simulink model "SS6_feb12"  (R2014b)
settings: Solver=ode3  StartTime=0.0  StopTime=40  FixedStep=0.001  RelTol=1e-3
undefined symbols (not defined in the file): INOP
libraries: simulink x1
settings Model: Creator=Bismaya  LastModifiedBy=Bismaya

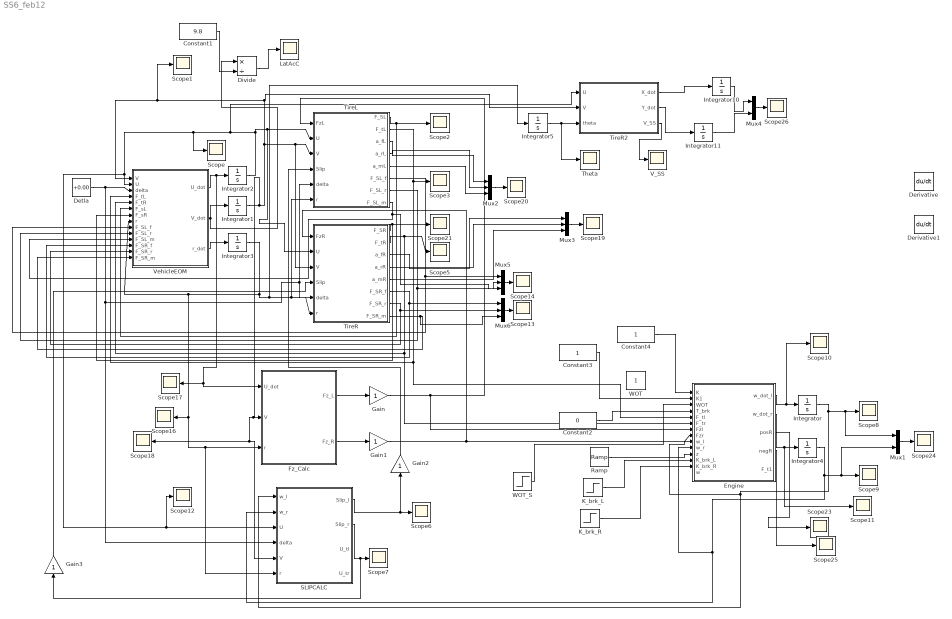
== system SS6_feb12 ==
  Constant1 : Constant  Value=9.8
  Constant2 : Constant  Value=0
  Constant3 : Constant
  Constant4 : Constant
  Derivative : Derivative
  Derivative1 : Derivative
  Detla : Constant  Value=+0.00
  Divide : Product  Inputs=*/
  Engine : MATLAB Function  TreatAsAtomicUnit=on
  Fz_Calc : MATLAB Function  TreatAsAtomicUnit=on
  Gain{,1..3} (4 alike) : Gain
  Integrator : Integrator  InitialCondition=12  LowerSaturationLimit=-0.0001
  Integrator{1,3,5,10..11} (5 alike) : Integrator
  Integrator2 : Integrator  InitialCondition=10/3
  Integrator4 : Integrator  InitialCondition=12  LowerSaturationLimit=-0.0001
  K_brk_L : Step  Time=0  After=0  SampleTime=0
  K_brk_R : Step  Time=20  After=INOP  SampleTime=0
  LatAcC : Scope
      settings: YMin=-2e-06  YMax=6e-06  SaveName=V1
  Mux1 : Mux  Inputs=2
  Mux{2..3,5..6} (4 alike) : Mux  Inputs=3
  Mux4 : Mux  Inputs=2
  Ramp : simulink/Sources/Ramp  slope=0  start=30  X0=2*13.5
  SLIPCALC : MATLAB Function  TreatAsAtomicUnit=on
  Scope{,1..3,5..14,16..21,23..26} (24 alike) : Scope
      Scope settings: YMin=20  YMax=45  SaveName=U
      Scope1 settings: YMin=-2e-06  YMax=6e-06  SaveName=V
      Scope10 settings: SaveName=ScopeData10
      Scope11 settings: SaveName=ScopeData11
      Scope12 settings: YMin=20  YMax=45  SaveName=ScopeData12
      Scope13 settings: YMin=20  YMax=45  SaveName=F_R
      Scope14 settings: YMin=20  YMax=45  SaveName=F_L
      Scope16 settings: YMin=20  YMax=45  SaveName=r
      Scope17 settings: YMin=20  YMax=45  SaveName=aX
      Scope18 settings: YMin=20  YMax=45  SaveName=ScopeData18
      Scope19 settings: YMin=20  YMax=45  SaveName=a_R  MaxDataPoints=5000000
      Scope2 settings: YMin=20  YMax=45  SaveName=F_SL
      Scope20 settings: YMin=20  YMax=45  SaveName=a_L  MaxDataPoints=5000000
      Scope21 settings: YMin=20  YMax=45  SaveName=F_SR  MaxDataPoints=5000000
      Scope24 settings: TimeRange=19.37  YMin=0  YMax=1500000000  SaveName=WheelSpeed
      Scope26 settings: YMin=20  YMax=45  SaveName=XY
      Scope3 settings: YMin=20  YMax=45  SaveName=F_tL  MaxDataPoints=5000000
      Scope5 settings: YMin=20  YMax=45  SaveName=F_tR
      Scope6 settings: TimeRange=40  YMin=26.58088235294118  YMax=36.58088235294118  SaveName=Slip_L
      Scope7 settings: TimeRange=7.18  YMin=0  YMax=1.4e+57  SaveName=Slip_R
      Scope8 settings: SaveName=ScopeData8
      Scope9 settings: YMin=-80  YMax=-20  SaveName=ScopeData9
  Theta : Scope
      settings: YMin=20  YMax=45  SaveName=Theta
  TireL : MATLAB Function  TreatAsAtomicUnit=on
  TireR : MATLAB Function  TreatAsAtomicUnit=on
  TireR2 : MATLAB Function  TreatAsAtomicUnit=on
  V_SS : Scope
      settings: YMin=20  YMax=45  SaveName=Theta1
  VehicleEOM : MATLAB Function  TreatAsAtomicUnit=on
  WOT : Constant
  "WOT_S " : Step  Time=0  Before=1  SampleTime=0
  wires:
  VehicleEOM/1(U_dot) -> Scope17/1, Fz_Calc/1(U_dot), Integrator2/1
  Integrator2/1 -> TireL/2(U), TireR/2(U), TireR2/1(U), Scope/1, Scope12/1, SLIPCALC/3(U), VehicleEOM/2(U)
  VehicleEOM/2(V_dot) -> Integrator1/1, Divide/1
  VehicleEOM/3(r_dot) -> Integrator3/1
  Integrator3/1 -> Integrator5/1, TireR/6(r), TireL/6(r), Scope16/1, SLIPCALC/6(r), Fz_Calc/3(r), VehicleEOM/8(r)
  Detla/1 -> SLIPCALC/4(delta), TireL/5(delta), TireR/5(delta), VehicleEOM/3(delta)
  SLIPCALC/2(Slip_r) -> Gain3/1, Scope7/1
  TireL/1(F_SL) -> VehicleEOM/6(F_sL), Scope2/1
  TireR/1(F_SR) -> VehicleEOM/7(F_sR), Scope21/1
  TireR/2(F_tR) -> Engine/6(F_tr), VehicleEOM/5(F_tR), Scope5/1
  Fz_Calc/1(Fz_L) -> Gain/1
  Fz_Calc/2(Fz_R) -> Gain1/1
  Gain/1 -> Engine/7(Fzl), TireL/1(FzL)
  Gain1/1 -> Engine/8(Fzr), TireR/1(FzR)
  Integrator/1 -> Mux1/1, Scope8/1, Engine/9(w_l), SLIPCALC/1(w_l)
  SLIPCALC/1(Slip_l) -> Gain2/1, Scope6/1
  Gain2/1 -> TireL/4(Slip)
  Gain3/1 -> TireR/4(Slip)
  Integrator4/1 -> Mux1/2, Scope9/1, Engine/10(w_r), SLIPCALC/2(w_r)
  "WOT_S "/1 -> Engine/3(WOT)
  TireL/2(F_tL) -> Scope3/1, Engine/5(F_tl), VehicleEOM/4(F_tL)
  Constant2/1 -> Engine/4(T_brk)
  Engine/1(w_dot_l) -> Scope10/1, Integrator/1
  Engine/2(w_dot_r) -> Scope11/1, Integrator4/1
  Integrator1/1 -> SLIPCALC/5(V), Scope18/1, Fz_Calc/2(V), TireR/3(V), TireL/3(V), TireR2/2(V), Scope1/1, VehicleEOM/1(V)
  Integrator5/1 -> TireR2/3(theta), Theta/1
  TireL/3(a_fL) -> Mux2/1
  TireR/3(a_fR) -> Mux3/1
  TireL/4(a_rL) -> Mux2/2
  TireR/4(a_rR) -> Mux3/2
  Constant3/1 -> Engine/2(K1)
  Mux1/1 -> Scope24/1
  Mux2/1 -> Scope20/1
  TireL/5(a_mL) -> Mux2/3
  Mux3/1 -> Scope19/1
  TireR/5(a_mR) -> Mux3/3
  Ramp/1 -> Engine/11(z)
  TireR2/1(X_dot) -> Integrator10/1
  TireR2/2(Y_dot) -> Integrator11/1
  Integrator11/1 -> Mux4/2
  Integrator10/1 -> Mux4/1
  Mux4/1 -> Scope26/1
  TireR/6(F_SR_f) -> Mux6/1, VehicleEOM/12(F_SR_f)
  TireR/7(F_SR_r) -> VehicleEOM/13(F_SR_r), Mux6/2
  TireL/8(F_SL_m) -> Mux5/3, VehicleEOM/11(F_SL_m)
  TireL/7(F_SL_r) -> Mux5/2, VehicleEOM/10(F_SL_r)
  TireL/6(F_SL_f) -> Mux5/1, VehicleEOM/9(F_SL_f)
  Mux5/1 -> Scope14/1
  TireR/8(F_SR_m) -> Mux6/3, VehicleEOM/14(F_SR_m)
  Mux6/1 -> Scope13/1
  Constant4/1 -> Engine/1(K)
  K_brk_R/1 -> Engine/13(K_brk_R)
  K_brk_L/1 -> Engine/12(K_brk_L)
  Engine/3(posR) -> Scope23/1
  Engine/4(negR) -> Scope25/1
  TireR2/3(V_SS) -> V_SS/1
  Constant1/1 -> Divide/2
  Divide/1 -> LatAcC/1

== matlab function SS6_feb12/TireL ==
  data: FzL input; F_SL output; F_tL output; U input; V input; Slip input; delta input; r input; a_fL output; a_rL output; a_mL output; F_SL_f output; F_SL_r output; F_SL_m output
function [F_SL,F_tL,a_fL,a_rL,a_mL,F_SL_f,F_SL_r,F_SL_m] = tireL(FzL,U,V,Slip,delta,r)
M=1280;Ms=1160;Izz=2500;Ixx=750;Ixz=0;a=1.203;b=1.217;hcg=0.5;e=0.2;Tw=1.33;R=0.3;I_t=2.1;
I_e=0.136;A_f=2.1;K_bf=0.55;zi1=13.56;z2=7.50;zi3=5.37;zi4=4.22;zi5=3.28;
Lbpsi=45000;Lbp=2600;C_a=20000;C_i=20000;mu=0.85;e_r=0.015;K_rsf=-0.05;K_rsr=0.1;
C1=-6.0;C2=59.16;C3=25;C_s1=1.38;K_rsf=0.444;C_d=0.32;d=0.014;n=0.85;
rho=1.204;g=9.81;c=0.2;


% FzF=M*g*mu/2;

Fz=FzL;

%Tire Longitudinal Velocity Calculation
% U_tf=U*cos(delta)+(V+a*r)*sin(delta);
% U_tr=U;
 U_tl=U+(0.5*Tw*r);
 U_tr=U-(0.5*Tw*r);
%FRONT Tires
 %Side Slip Calc
a_fL=-atan((V+a*r)/(U+0.5*Tw*r));
a_rL=atan((b*r-V)/(U+0.5*Tw*r));
a_mL=atan((c*r-V)/(U+0.5*Tw*r));

alpha=a_fL;
%Tire Equations
S_f=(mu*(Fz/3)*(1-(e_r*U_tl*sqrt((Slip*Slip)+(tan(alpha)*tan(alpha)))))*(1-Slip))/...
    (2*sqrt(C_i*C_i*Slip*Slip+C_a*C_a*tan(alpha)*tan(alpha)));
if(S_f<1)
    f_S=S_f*(2-S_f);
else
    f_S=1;
end
F_SL_f=(C_a*tan(alpha)*f_S)/(1-Slip);
F_tL_f=(C_i*Slip*f_S)/(1-Slip);

%Rear Tires
alpha=a_rL;

S_r=(mu*(Fz/3)*(1-(e_r*U_tl*sqrt((Slip*Slip)+(tan(alpha)*tan(alpha)))))*(1-Slip))/...
    (2*sqrt(C_i*C_i*Slip*Slip+C_a*C_a*tan(alpha)*tan(alpha)));
if(S_r<1)
    f_S=S_r*(2-S_r);
else
    f_S=1;
end
F_SL_r=(C_a*tan(alpha)*f_S)/(1-Slip);
F_tL_r=(C_i*Slip*f_S)/(1-Slip);

%Middle Tires
alpha=a_mL;

S_m=(mu*(Fz/3)*(1-(e_r*U_tl*sqrt((Slip*Slip)+(tan(alpha)*tan(alpha)))))*(1-Slip))/...
    (2*sqrt(C_i*C_i*Slip*Slip+C_a*C_a*tan(alpha)*tan(alpha)));
if(S_m<1)
    f_S=S_m*(2-S_m);
else
    f_S=1;
end
F_SL_m=(C_a*tan(alpha)*f_S)/(1-Slip);
F_tL_m=(C_i*Slip*f_S)/(1-Slip);


F_SL=F_SL_f+F_SL_r+F_SL_m;
F_tL=F_tL_f+F_tL_r+F_tL_m;
F_L=[F_tL_f;F_tL_r;F_tL_m;F_SL_f;F_SL_r;F_SL_m;];

== matlab function SS6_feb12/Engine ==
  data: K input; K1 input; WOT input; T_brk input; F_tl input; F_tr input; Fzl input; Fzr input; w_l input; w_r input; w_dot_l output; w_dot_r output; posR output; negR output; z input; F_t1 output; K_brk_L input; K_brk_R input; w input
function [w_dot_l,w_dot_r,posR,negR,F_t1] = fcn(K,K1,WOT,T_brk,F_tl,F_tr,Fzl,Fzr,w_l,w_r,z,K_brk_L,K_brk_R,w)
M=1280;Ms=1160;Izz=2500;Ixx=750;Ixz=0;a=1.203;b=1.217;hcg=0.5;e=0.2;Tw=1.33;R=0.3;I_t=2.1;
I_e=0.136;A_f=2.1;zi1=2.5*13.56;zi2=7.50;zi3=5.37;zi4=4.22;zi5=3.28;
Lbpsi=45000;Lbp=2600;C_a=20000;C_i=20000;mu=0.85;e_r=0.015;K_rsf=-0.05;K_rsr=0.1;
C1=-6.0;C2=59.16;C3=25;C_s1=1.38;K_rsf=0.444;C_d=0.32;d=0.014;n=0.85;
rho=1.204;g=9.81;
K_bf=0.55;
zi=z;

% Fzf=M*g/2;
% Fzr=M*g/2;
F_tl=F_tl;
F_tr=F_tr;
F_t1=F_tl+F_tr;
%Engine Equations
w_el=zi*K1*w_l;
w_er=zi*K*w_r;

% w_el=400;
% w_er=400;

IwL=I_t+(0.5*K1*K1*zi*zi*n*I_e);%Accelerating
IwR=I_t+(0.5*K*K*zi*zi*n*I_e);%Accelerating
% IwL=1.5*IwL;
% IwR=1.5*IwR;
T_l=WOT*zi*K1*n*(C1*(w_el/100)^2+C2*(w_el/100)+C3);
T_r=WOT*zi*K*n*(C1*(w_er/100)^2+C2*(w_er/100)+C3);
T_trac_L=T_l-(R*F_tl)-(d*Fzl);
T_trac_R=T_r-(R*F_tr)-(d*Fzr);
T_brkl=K_brk_L*T_l;
T_brkr=K_brk_R*T_r;
w_dot_l=(1/(IwL))*(T_trac_L-T_brkl);
w_dot_r=(1/(IwR))*(T_trac_R-T_brkr);
% w_dot_f=(1/Iw)*(T_f-(d*Fzf)-(0.5*T_brkf));
% w_dot_r=(1/Iw)*(T_r-(d*Fzr)-(0.5*T_brkr));
% posR=T_l;
posR=T_trac_L;

% negR=(R*F_tr)+(d*Fzr)+(0.5*T_brkr);
negR=w_dot_l;
posL=T_l;
negL=(R*F_tl)+(d*Fzl)+(0.5*T_brkl);

== matlab function SS6_feb12/TireR ==
  data: FzR input; F_SR output; F_tR output; U input; V input; Slip input; delta input; r input; a_fR output; a_rR output; a_mR output; F_SR_f output; F_SR_r output; F_SR_m output
function [F_SR,F_tR,a_fR,a_rR,a_mR,F_SR_f,F_SR_r,F_SR_m] = tireR(FzR,U,V,Slip,delta,r)
M=1280;Ms=1160;Izz=2500;Ixx=750;Ixz=0;a=1.203;b=1.217;hcg=0.5;e=0.2;Tw=1.33;R=0.3;I_t=2.1;
I_e=0.136;A_f=2.1;K_bf=0.55;zi1=13.56;z2=7.50;zi3=5.37;zi4=4.22;zi5=3.28;
Lbpsi=45000;Lbp=2600;C_a=20000;C_i=20000;mu=0.85;e_r=0.015;K_rsf=-0.05;K_rsr=0.1;
C1=-6.0;C2=59.16;C3=25;C_s1=1.38;K_rsf=0.444;C_d=0.32;d=0.014;n=0.85;
rho=1.204;g=9.81;c=0.2;


% FzF=M*g*mu/2;
Fz=FzR;

%Tire Longitudinal Velocity Calculation
% U_tf=U*cos(delta)+(V+a*r)*sin(delta);
% U_tr=U;

 %Side Slip Calc
a_fR=-atan((V+a*r)/(U-0.5*Tw*r));
a_rR=atan((b*r-V)/(U-0.5*Tw*r));
a_mR=atan((c*r-V)/(U-0.5*Tw*r));

alpha=a_fR;

 U_tl=U+(0.5*Tw*r);
 U_tr=U-(0.5*Tw*r);
%%FRONT Tires
%Tire Equations
S_f=(mu*(Fz/3)*(1-(e_r*U_tr*sqrt((Slip*Slip)+(tan(alpha)*tan(alpha)))))*(1-Slip))/...
    (2*sqrt(C_i*C_i*Slip*Slip+C_a*C_a*tan(alpha)*tan(alpha)));
if(S_f<1)
    f_S=S_f*(2-S_f);
else
    f_S=1;
end
F_SR_f=(C_a*tan(alpha)*f_S)/(1-Slip);
F_tR_f=(C_i*Slip*f_S)/(1-Slip);

%%Rear Tires
alpha=a_rR;

S_r=(mu*(Fz/3)*(1-(e_r*U_tr*sqrt((Slip*Slip)+(tan(alpha)*tan(alpha)))))*(1-Slip))/...
    (2*sqrt(C_i*C_i*Slip*Slip+C_a*C_a*tan(alpha)*tan(alpha)));
if(S_r<1)
    f_S=S_r*(2-S_r);
else
    f_S=1;
end
F_SR_r=(C_a*tan(alpha)*f_S)/(1-Slip);
F_tR_r=(C_i*Slip*f_S)/(1-Slip);

%%Middle Tires
alpha=a_mR;

S_m=(mu*(Fz/3)*(1-(e_r*U_tr*sqrt((Slip*Slip)+(tan(alpha)*tan(alpha)))))*(1-Slip))/...
    (2*sqrt(C_i*C_i*Slip*Slip+C_a*C_a*tan(alpha)*tan(alpha)));
if(S_m<1)
    f_S=S_m*(2-S_m);
else
    f_S=1;
end
F_SR_m=(C_a*tan(alpha)*f_S)/(1-Slip);
F_tR_m=(C_i*Slip*f_S)/(1-Slip);


F_SR=F_SR_f+F_SR_r+F_SR_m;
F_tR=F_tR_f+F_tR_r+F_tR_m;
F_R=[F_tR_f;F_tR_r;F_tR_m;F_SR_f;F_SR_r;F_SR_m];

== matlab function SS6_feb12/VehicleEOM ==
  data: V input; U_dot output; V_dot output; U input; delta input; F_tL input; F_tR input; F_sL input; F_sR input; r_dot output; r input; F_SL_f input; F_SL_r input; F_SL_m input; F_SR_f input; F_SR_r input; F_SR_m input
function [U_dot,V_dot,r_dot] = VehicleEOM(V,U,delta,F_tL,F_tR,F_sL,F_sR,r,F_SL_f,F_SL_r,F_SL_m,F_SR_f,F_SR_r,F_SR_m)
M=1280;Ms=1160;Izz=2500;Ixx=750;Ixz=0;a=1.203;b=1.217;hcg=0.5;e=0.2;Tw=1.33;R=0.3;I_t=2.1;
I_e=0.136;A_f=2.1;K_bf=0.55;zi1=13.56;z2=7.50;zi3=5.37;zi4=4.22;zi5=3.28;
Lbpsi=45000;Lbp=2600;C_a=20000;C_i=20000;mu=0.85;e_r=0.015;K_rsf=-0.05;K_rsr=0.1;
C1=-6.0;C2=59.16;C3=25;C_s1=1.38;K_rsf=0.444;C_d=0.32;d=0.014;n=0.85;
rho=1.204;g=9.81;c=0.2;

F_t=(F_tL+F_tR);
%Vehicle Equations
% U_dot=(1/M)*((M*V*r)+F_t-(0.5*C_d*A_f*rho*U*U));
U_dot=(1/M)*((M*V*r)+F_t);

V_dot=(1/M)*((-M*U*r)+F_sL+F_sR);
% r_dot=(1/Izz)*(2*a*F_tL*sin(delta)+2*a*F_sL*cos(delta)-2*b*F_sR);
 r_dot=(1/(0.5*Izz))*(0.5*Tw*F_tL-0.5*Tw*F_tR+a*(F_SL_f+F_SR_f)-b*(F_SL_r+F_SR_r)-c*(F_SL_m+F_SR_m));

== matlab function SS6_feb12/SLIPCALC ==
  data: w_l input; w_r input; Slip_l output; Slip_r output; U input; delta input; V input; r input; U_tl output; U_tr output
function [Slip_l,Slip_r,U_tl,U_tr] = SlipCalc(w_l,w_r,U,delta,V,r)
M=1280;Ms=1160;Izz=2500;Ixx=750;Ixz=0;a=1.203;b=1.217;hcg=0.5;e=0.2;Tw=1.33;R=0.3;I_t=2.1;
I_e=0.136;A_f=2.1;K_bf=0.55;zi1=13.56;z2=7.50;zi3=5.37;zi4=4.22;zi5=3.28;
Lbpsi=45000;Lbp=2600;C_a=20000;C_i=20000;mu=0.85;e_r=0.015;K_rsf=-0.05;K_rsr=0.1;
C1=-6.0;C2=59.16;C3=25;C_s1=1.38;K_rsf=0.444;C_d=0.32;d=0.014;n=0.85;
rho=1.204;g=9.81;

% w_r=-w_r;
% w_f=-w_f;
%Tire Longitudinal Velocity Calculation
% U_tl=U*cos(delta)+(V+a*r)*sin(delta);
% U_tr=U;
 U_tl=U+(0.5*Tw*r);
 U_tr=U-(0.5*Tw*r);

% %  SlipCalc
% if(U_tl<=(R*w_l))
%     Slip_l=1-(U_tl/(R*w_l));%Acceleration
% else
%     Slip_l=1-((R*w_l)/U_tl);%Braking
% %     Slip_l=0;
% end
% 
% if(U_tr<=(R*w_r))
%     Slip_r=1-(U_tr/(R*w_r));%Acceleration
% else
%     Slip_r=1-((R*w_r)/U_tr);%Braking
% %     Slip_r=0;
% end
Slip_l=1-(U_tl/(R*w_l));
Slip_r=1-(U_tr/(R*w_r));

% 
% if(Slip_l<0)
%      Slip_l=0;
%  elseif (Slip_l>1)
%          Slip_l=1;
%  end
%  if(Slip_r<0)
%      Slip_r=0;
%  elseif (Slip_r>1)
%          Slip_r=1;
%  end
% %

== matlab function SS6_feb12/Fz_Calc ==
  data: U_dot input; V input; Fz_L output; Fz_R output; r input
function [Fz_L,Fz_R] = FzCalc(U_dot,V,r)
M=1280;Ms=1160;Izz=2500;Ixx=750;Ixz=0;a=1.203;b=1.217;hcg=0.5;e=0.2;Tw=1.33;R=0.3;I_t=2.1;
I_e=0.136;A_f=2.1;K_bf=0.55;zi1=13.56;z2=7.50;zi3=5.37;zi4=4.22;zi5=3.28;
Lbpsi=45000;Lbp=2600;C_a=20000;C_i=20000;mu=0.85;e_r=0.015;K_rsf=-0.05;K_rsr=0.1;
C1=-6.0;C2=59.16;C3=25;C_s1=1.38;K_rsf=0.444;C_d=0.32;d=0.014;n=0.85;
rho=1.204;g=9.81;


%NormalForceCalc
% Fz_f=(M*g/2)*((b/(a+b))-((U_dot-V*r)*hcg)/(g*(a+b)));
% Fz_r=(M*g/2)*((a/(a+b))+((U_dot-V*r)*hcg)/(g*(a+b)));
Fz_L=(M*g/2);
Fz_R=(M*g/2);

== matlab function SS6_feb12/TireR2 ==
  data: U input; V input; theta input; X_dot output; Y_dot output; V_SS output
function [X_dot,Y_dot, V_SS] = CT(U,V,theta)
M=1280;Ms=1160;Izz=2500;Ixx=750;Ixz=0;a=1.203;b=1.217;hcg=0.5;e=0.2;Tw=1.33;R=0.3;I_t=2.1;
I_e=0.136;A_f=2.1;K_bf=0.55;zi1=13.56;z2=7.50;zi3=5.37;zi4=4.22;zi5=3.28;
Lbpsi=45000;Lbp=2600;C_a=20000;C_i=20000;mu=0.85;e_r=0.015;K_rsf=-0.05;K_rsr=0.1;
C1=-6.0;C2=59.16;C3=25;C_s1=1.38;K_rsf=0.444;C_d=0.32;d=0.014;n=0.85;
rho=1.204;g=9.81;c=0.2;

X_dot=U*cos(theta)-V*sin(theta);
Y_dot=+U*sin(theta)+V*cos(theta);
V_SS=atand(V/U);
